simulink model "Bagimport"  (R2017b)
settings: Solver=VariableStepAuto  StartTime=0.0  StopTime=10.0  RelTol=1e-3
libraries: robotlib x1
settings Model: Creator=mccla  LastModifiedBy=mccla

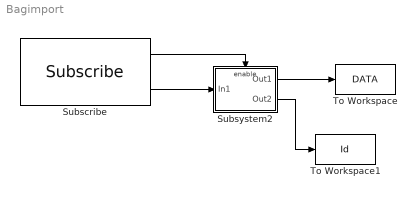
== system Bagimport ==
  Subscribe : robotlib/Subscribe  SourceLibraryInfo=This block requires Robotics System Toolbox  topicSource=Specify your own  topic=/tag_detections  messageType=apriltags2_ros/AprilTagDetectionArray  sampleTime=-1  messageQueueLength=1
      settings: SourceProductBaseCode=RO
  Subsystem2 : Subsystem
  To Workspace : ToWorkspace  VariableName=DATA  SaveFormat=Timeseries  SampleTime=-1
  To Workspace1 : ToWorkspace  VariableName=Id  SaveFormat=Timeseries  SampleTime=-1
  wires:
  Subscribe/2 -> Subsystem2/1(In1)
  Subscribe/1 -> Subsystem2/Enable
  Subsystem2/1(Out1) -> To Workspace/1
  Subsystem2/2(Out2) -> To Workspace1/1

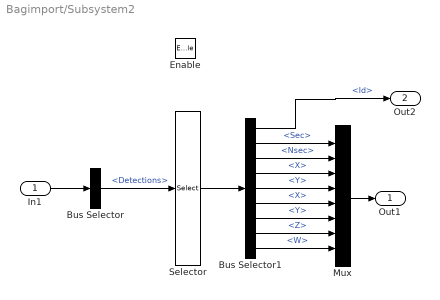
== system Bagimport/Subsystem2 ==
  In1 : Inport
  Enable : EnablePort
  Bus Selector : BusSelector  OutputSignals=Detections
  Bus Selector1 : BusSelector  OutputSignals=Id,Pose.Header.Stamp.Sec,Pose.Header.Stamp.Nsec,Pose.Pose.Pose.Position.X,Pose.Pose.Pose.Position.Y,Pose.Pose.Pose.Orientation.X,Pose.Pose.Pose.Orientation.Y,Pose.Pose.Pose.Orientation.Z,Pose.Pose.Pose.Orientation.W
  Mux : Mux  Inputs=8
  Selector : Selector  InputPortWidth=16  IndexOptions=Index vector (dialog)  Indices=[2]  OutputSizes=1
  Out1 : Outport
  Out2 : Outport  Port=2
  wires:
  Selector/1 -> Bus Selector1/1
  Bus Selector/1 -> Selector/1  "<Detections>"
  In1/1 -> Bus Selector/1
  Bus Selector1/2 -> Mux/1  "<Sec>"
  Bus Selector1/3 -> Mux/2  "<Nsec>"
  Bus Selector1/4 -> Mux/3  "<X>"
  Bus Selector1/5 -> Mux/4  "<Y>"
  Bus Selector1/6 -> Mux/5  "<X>"
  Bus Selector1/7 -> Mux/6  "<Y>"
  Bus Selector1/8 -> Mux/7  "<Z>"
  Bus Selector1/9 -> Mux/8  "<W>"
  Mux/1 -> Out1/1
  Bus Selector1/1 -> Out2/1  "<Id>"
